simulink model "III_ph_VSI"  (R2022a)
settings: Solver=VariableStepAuto  StartTime=0.0  StopTime=0.1  RelTol=1e-3
InitFcn:
  | Vdc=150;
settings Model: Creator=darsh  LastModifiedBy=darsh

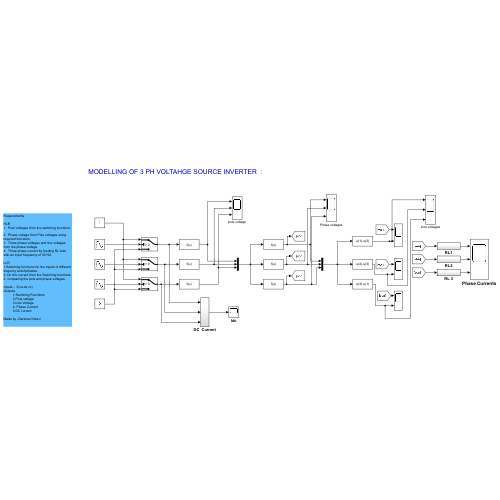
[thumbnail: Simulink's stored preview of the top-level diagram]
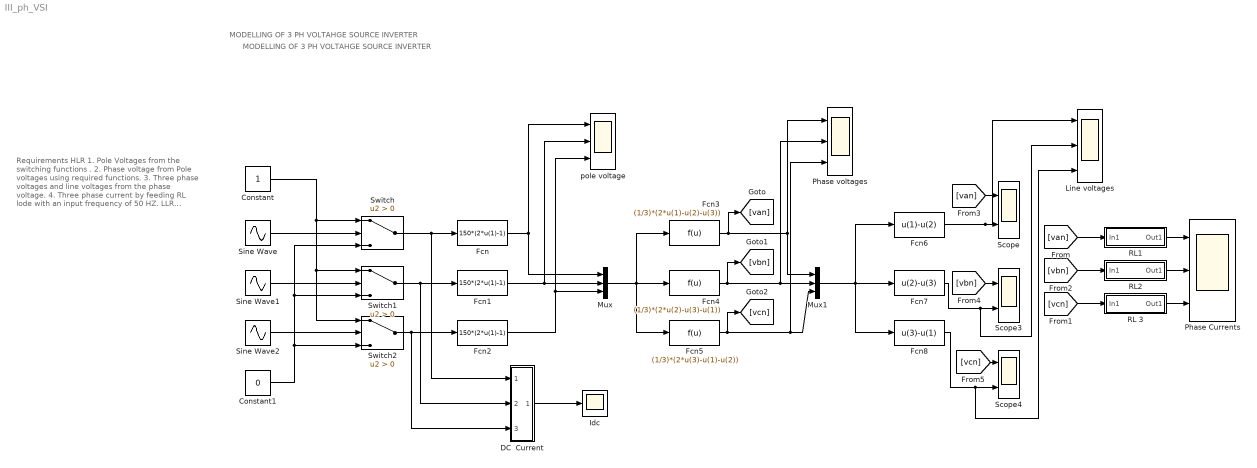
== system III_ph_VSI ==
  note: Requirements
      |
      | HLR
      | 1. Pole Voltages from the switching functions .
      | 2. Phase voltage from Pole voltages using required functions.
      | 3. Three phase voltages and line voltages from the phase voltage.
      | 4. Three phase current by feeding RL lode with an input frequency of 50 HZ.
      |
      | LLR
      | 1.Switching functions for the inputs of different frequncy and Aplitudes.
      | 2. Dc link current from the Switching functions.
      | 3. comparing the pole and phase voltages.
      |
      | Inputs - 3(va,vb,vc)
      | Outputs
      | 1.Switching Functions
      | 2.Pole voltage
      | 3.Line Voltage
      | 4. Phase Current
      | 5.DC current.
      |
      | Made by -Darshan Kolavi
  note: MODELLING OF 3 PH VOLTAHGE SOURCE INVERTER
  note: MODELLING OF 3 PH VOLTAHGE SOURCE INVERTER
  Constant : Constant
  Constant1 : Constant  Value=0
  DC  Current : Subsystem
  Fcn : Fcn  Expr=150*(2*u(1)-1)
  Fcn1 : Fcn  Expr=150*(2*u(1)-1)
  Fcn2 : Fcn  Expr=150*(2*u(1)-1)
  Fcn3 : Fcn  Expr=(1/3)*(2*u(1)-u(2)-u(3))
  Fcn4 : Fcn  Expr=(1/3)*(2*u(2)-u(3)-u(1))
  Fcn5 : Fcn  Expr=(1/3)*(2*u(3)-u(1)-u(2))
  Fcn6 : Fcn  Expr=u(1)-u(2)
  Fcn7 : Fcn  Expr=u(2)-u(3)
  Fcn8 : Fcn  Expr=u(3)-u(1)
  Idc : Scope
  Line voltages : Scope  NumInputPorts=3
  Mux : Mux  Inputs=3
  Mux1 : Mux  Inputs=3
  Phase Currents : Scope  NumInputPorts=3
  Phase voltages : Scope  NumInputPorts=3
  RL 3 : Subsystem
  RL1 : Subsystem
  RL2 : Subsystem
  Scope : Scope  NumInputPorts=2
  Scope3 : Scope  NumInputPorts=2
  Scope4 : Scope  NumInputPorts=2
  Sine Wave : Sin  Frequency=314.16  SampleTime=0
  Sine Wave1 : Sin  Amplitude=2  Frequency=314.16  Phase=-2.095  SampleTime=0
  Sine Wave2 : Sin  Frequency=314.16  Phase=-4.189  SampleTime=0
  Switch : Switch  Criteria=u2 > Threshold  SaturateOnIntegerOverflow=off  InputSameDT=off
  Switch1 : Switch  Criteria=u2 > Threshold  SaturateOnIntegerOverflow=off  InputSameDT=off
  Switch2 : Switch  Criteria=u2 > Threshold  SaturateOnIntegerOverflow=off  InputSameDT=off
  pole voltage : Scope  NumInputPorts=3
  wires:
  Mux/1 -> Fcn4/1, Fcn5/1, Fcn3/1
  Constant1/1 -> Switch/3, Switch1/3, Switch2/3
  Sine Wave/1 -> Switch/2
  Fcn3/1 -> Phase voltages/1, Mux1/1, [van]
  Fcn1/1 -> pole voltage/2, Mux/2
  Fcn8/1 -> Line voltages/3, Scope4/2
  Switch/1 -> DC  Current/1(In1), Fcn/1
  [vcn] -> Scope4/1
  [van] -> Scope/1
  Fcn7/1 -> Line voltages/2, Scope3/2
  Switch2/1 -> Fcn2/1, DC  Current/3(In3)
  [vbn] -> RL2/1(In1)
  RL1/1(Out1) -> Phase Currents/1
  RL2/1(Out1) -> Phase Currents/2
  Sine Wave1/1 -> Switch1/2
  Fcn5/1 -> Phase voltages/3, Mux1/3, [vcn]
  [vcn] -> RL 3/1(In1)
  [van] -> RL1/1(In1)
  [vbn] -> Scope3/1
  RL 3/1(Out1) -> Phase Currents/3
  Constant/1 -> Switch1/1, Switch2/1, Switch/1
  Fcn2/1 -> pole voltage/3, Mux/3
  DC  Current/1(Out1) -> Idc/1
  Switch1/1 -> Fcn1/1, DC  Current/2(In2)
  Mux1/1 -> Fcn8/1, Fcn6/1, Fcn7/1
  Fcn4/1 -> Phase voltages/2, Mux1/2, [vbn]
  Fcn/1 -> pole voltage/1, Mux/1
  Fcn6/1 -> Line voltages/1, Scope/2
  Sine Wave2/1 -> Switch2/2

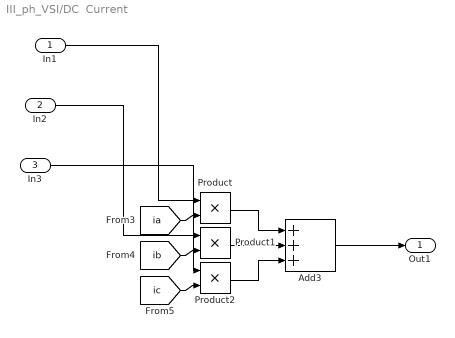
== system III_ph_VSI/DC  Current ==
  In1 : Inport
  In2 : Inport  Port=2
  In3 : Inport  Port=3
  Add3 : Sum  Inputs=+++
  Product : Product
  Product1 : Product
  Product2 : Product
  Out1 : Outport  VectorParamsAs1DForOutWhenUnconnected=off
  wires:
  [ic] -> Product2/2
  [ib] -> Product1/2
  [ia] -> Product/2
  Add3/1 -> Out1/1
  Product/1 -> Add3/1
  In3/1 -> Product2/1
  Product2/1 -> Add3/3
  In1/1 -> Product/1
  Product1/1 -> Add3/2
  In2/1 -> Product1/1

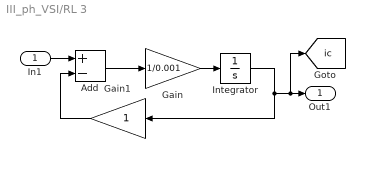
== system III_ph_VSI/RL 3 ==
  In1 : Inport
  Add : Sum  Inputs=+-
  Gain : Gain  Gain=1/0.001
  Gain1 : Gain
  Integrator : Integrator
  Out1 : Outport  VectorParamsAs1DForOutWhenUnconnected=off
  tag scope: ic=global
  wires:
  In1/1 -> Add/1
  Integrator/1 -> [ic], Out1/1, Gain1/1
  Gain1/1 -> Add/2
  Gain/1 -> Integrator/1
  Add/1 -> Gain/1

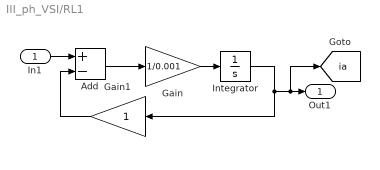
== system III_ph_VSI/RL1 ==
  In1 : Inport
  Add : Sum  Inputs=+-
  Gain : Gain  Gain=1/0.001
  Gain1 : Gain
  Integrator : Integrator
  Out1 : Outport  VectorParamsAs1DForOutWhenUnconnected=off
  tag scope: ia=global
  wires:
  In1/1 -> Add/1
  Integrator/1 -> [ia], Out1/1, Gain1/1
  Gain1/1 -> Add/2
  Gain/1 -> Integrator/1
  Add/1 -> Gain/1

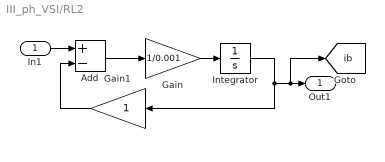
== system III_ph_VSI/RL2 ==
  In1 : Inport
  Add : Sum  Inputs=+-
  Gain : Gain  Gain=1/0.001
  Gain1 : Gain
  Integrator : Integrator
  Out1 : Outport  VectorParamsAs1DForOutWhenUnconnected=off
  tag scope: ib=global
  wires:
  In1/1 -> Add/1
  Integrator/1 -> [ib], Out1/1, Gain1/1
  Gain1/1 -> Add/2
  Gain/1 -> Integrator/1
  Add/1 -> Gain/1
